simulink model "Dynamic_mini_project"  (R2022b)
settings: Solver=VariableStepAuto  StartTime=0.0  StopTime=1.0  FixedStep=0.0001  RelTol=1e-3  EnableMultiTasking=on
settings Model: Creator=shb  LastModifiedBy=Jakob Jørgensen
settings SolverCC: AlgebraicLoopSolver=TrustRegion
settings DataIOCC: LimitDataPoints=on  SaveFormat=Array  ReturnWorkspaceOutputs=off
settings OptimizationCC: LifeSpan=inf
settings DebuggingCC: UnconnectedInputMsg=warning  UnconnectedOutputMsg=warning  UnconnectedLineMsg=warning  SFUnexpectedBacktrackingDiag=warning  SFNoUnconditionalDefaultTransitionDiag=warning  SFExecutionAtInitializationDiag=none  SFMachineParentedDataDiag=warning  ArithmeticOperatorsInVariantConditions=warning
settings HardwareCC: ProdBitPerPointer=32  ProdBitPerSizeT=32  ProdBitPerPtrDiffT=32  ProdLargestAtomicFloat=None  ProdIntDivRoundTo=Undefined  ProdEndianess=Unspecified  ProdWordSize=32  ProdHWDeviceType=32-bit Generic
settings ModelReferenceCC: EnableRefExpFcnMdlSchedulingChecks=on  PropagateSignalLabelsOutOfModel=off
settings SFSimCC: SimUseLocalCustomCode=off  CustomCodeUndefinedFunction=UseInterfaceOnly
settings RTWCC: RTWUseLocalCustomCode=off  DLArmComputeVersion=19.05
settings CodeAppCC: StateflowObjectComments=on
settings GRTTargetCC: TargetLangStandard=C89/C90 (ANSI)
settings ConfigComp: CovMetricSettings=dw  CovSaveCumulativeToWorkspaceVar=on  CovSaveSingleToWorkspaceVar=on  CovExternalEMLEnable=off

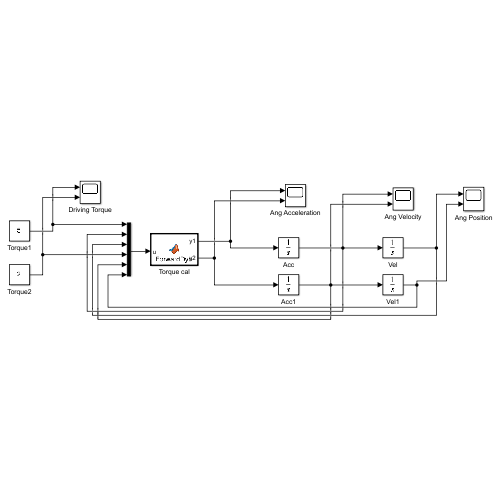
[thumbnail: Simulink's stored preview of the top-level diagram]
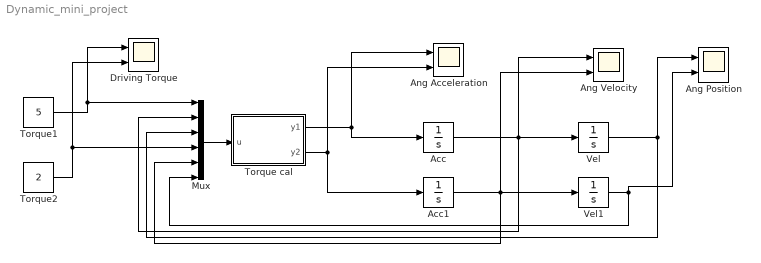
== system Dynamic_mini_project ==
  Acc : Integrator
  Acc1 : Integrator
  Ang Acceleration : Scope  NumInputPorts=2
  Ang Position : Scope  NumInputPorts=2
  Ang Velocity : Scope  NumInputPorts=2
  Driving Torque : Scope  NumInputPorts=2
  Mux : Mux  Inputs=6
  Torque cal : MATLAB Function  TreatAsAtomicUnit=on
  Torque1 : Constant  Value=5
  Torque2 : Constant  Value=2
  Vel : Integrator
  Vel1 : Integrator
  wires:
  Torque1/1 -> Driving Torque/1, Mux/1
  Mux/1 -> Torque cal/1(u)
  Torque cal/1(y1) -> Acc/1, Ang Acceleration/1
  Acc/1 -> Ang Velocity/1, Mux/2, Vel/1
  Vel/1 -> Mux/3, Ang Position/1
  Torque2/1 -> Driving Torque/2, Mux/4
  Torque cal/2(y2) -> Acc1/1, Ang Acceleration/2
  Acc1/1 -> Mux/5, Vel1/1, Ang Velocity/2
  Vel1/1 -> Mux/6, Ang Position/2

== matlab function Dynamic_mini_project/Torque cal ==
  data: u input; y1 output; y2 output
function [y1,y2]= ForwardDyn(u)

%%   motor torques
tau_1 = u(1);
tau_2 = u(4);

%% joint velocity and displacement
 theta_1 = u(3);  theta_2 = u(6);
 %dtheta_2 =u(5);dtheta_1 = u(2); 

%%  %%%%%%%%%%%%%%%%%%%%%%%  motion profiles
% %=======================  joint 1
% A1 = 0.3; % magnitude
% f1 = 5; % frequency
% 
% %=======================  joint 2
% A2 = 0.5; % magnitude
% f2 = 2; % frequency

g = 9.801; % gravity constant 
rho = 7806; 
%% %%%%%%%%%%%%%%%%%%%%%%%%%%%%  link 1 properties
%======================================  link 1
L1 = 1; % length [m]
c1 = L1/2; % mass center
m1 = L1*0.05*0.05*rho; % mass [kg]
I1 = 1/12*m1*L1^2; % moment of inertia


%% %%%%%%%%%%%%%%%%%%%%%%%%%%%%  link 2 properties
%======================================  link 2
L2 = 0.5; % length [m]
c2 = L2/2; % mass center
m2 = L2*0.05*0.05*rho; % mass [kg]
I2 = 1/12*m2*L2^2; % moment of inertia

%% %%%%%%%%%%%%%%%%%% dynamic simulation

    %%%%%%%%%%%%%%%%%%%%%%%%%%%  coefficients of dynamic equation
    H1 = m1*c1^2 + I1+I2+m2*(L1^2+c2^2+2*L1*c2*cos(theta_2)); 
    H2 = m1*c2^2+I2; 
    G1 = m1*g*(c1*cos(theta_1))+m2*g*(L1*cos(theta_1)+c2*cos(theta_1+theta_2));
    G2 = m1*c1*g*cos(theta_1+theta_2);  
    
%     %%%%%%%%%%%%%%%%%%%%%%%%%%%%%%%%%%%%%  actuator torques
%     tau_1 = H11*ddtheta_1 + H12*ddtheta_2 - h*(dtheta_2)^2 ...
%         -2*h*dtheta_1*dtheta_2 + G1;
%     tau_2 = H22*ddtheta_2 + H12*ddtheta_1 + h*(dtheta_1)^2 + G2;
    
    torque1 = tau_1 + G1; 
    torque2 = tau_2 + G2; 
    y1 = H1\torque1;  
    y2 = H2\torque2;
